simulink model "process_viewer_1"  (R2016b)
settings: Solver=VariableStepAuto  StartTime=0.0  StopTime=10.0  RelTol=1e-3
values from neighbouring files (symbols this model uses):
  frames = frames_full.Array_of_data(range)    [code.m]    (also in code_11111111111111111111111111.m = frames_full.Array_of_data())
settings Model: Creator=Ignat  LastModifiedBy=Ignat

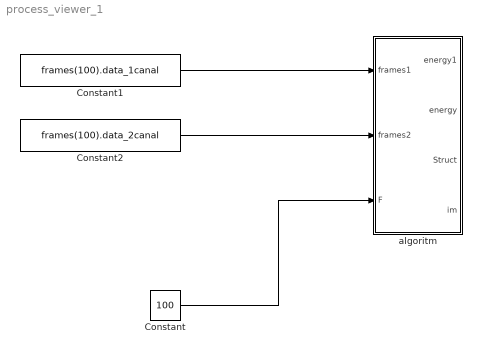
== system process_viewer_1 ==
  Constant : Constant  Value=100
  Constant1 : Constant  Value=frames(100).data_1canal
  Constant2 : Constant  Value=frames(100).data_2canal
  algoritm : MATLAB Function  TreatAsAtomicUnit=on
  wires:
  Constant/1 -> algoritm/3(F)
  Constant1/1 -> algoritm/1(frames1)
  Constant2/1 -> algoritm/2(frames2)

== matlab function process_viewer_1/algoritm ==
  data: frames1 input; frames2 input; energy1 output; energy output; Struct output; im output; F input
function [energy1,energy,Struct,im] = fcn(frames1,frames2,F)
ss1 = double(frames1);
ss2 = double(frames2);
EQ256 = 256; % число, эквивалентное 256
EQ64 = 64; % число, эквивалентное 64
Rd = 3;  %разрешение по дальности
Vd = 0.78125; %разрешение по скорости
BufferIn1 = ss1';
BufferIn2 = ss2';

% БПФ с прореживанием по времени
BufferFFTt1 = fft(BufferIn1);
BufferFFTt2 = fft(BufferIn2);

%отсечка симметричной части
%преобразуем [256][64] в [128][64]
BufferFFTt1(EQ256/2+1:EQ256,:) = [];
BufferFFTt2(EQ256/2+1:EQ256,:) = [];

% операция транспонирования матрицы
BufferFFTt1 = BufferFFTt1';
BufferFFTt2 = BufferFFTt2';

% БПФ с прореживанием по частоте    
BufferFFTw1 = fft(BufferFFTt1);
BufferFFTw2 = fft(BufferFFTt2);

% расчет мощности в каждой точке (сумма модулей соответствующих двух чисел)
energy0 = abs(BufferFFTw1) + abs(BufferFFTw2);
% преобразование матрица дальность-скорость к "привычному" виду
energy1(1:1:32,:) = energy0(32:-1:1,:);
energy1(33:1:64,:) = energy0(64:-1:33,:);

k = 6; % коэффициент порога
n_look = 3; % колличество обозреваемых точек 
n_miss = 2; % колличество пропускаемых точек 

% пороговая фильтрация
energy = threshold_filter(energy1, k, EQ64, EQ256/2, n_look, n_miss);

% расчет угла
arg = argument(BufferIn1, BufferIn2, energy, EQ64, EQ256/2);

% кластеризация и заполнение структуры
% нулевая скорость в 32 строке energy -> 64 строка неинформативна
Struct = clustering(energy, energy1, arg, Rd, Vd, EQ64, EQ256/2);

ax = Rd:Rd:128*Rd;
ay = -31*Vd:Vd:32*Vd;
im = image(ax,ay, energy1, 'CDataMapping' , 'scaled' );
